simulink model "kde"  (R2022b)
settings: Solver=VariableStepAuto  StartTime=0.0  StopTime=orbit_E.T  RelTol=1e-9
values from neighbouring files (symbols this model uses):
  A0 = [1 0 0; 0 1 0; 0 0 1]    [test_script.m]
  earth_horizon = struct('dvst', 3*0.2 ,'accuracy', deg2rad(0.2))    [test_script.m]
  gyro = struct('c', 15e-3, 'ARW', 0.15, 'sigma_b', deg2rad(0.3) / 3600,                'freq', 262, 'accuracy', 2.4e-9)    [test_script.m]
  H0 = sqrt((-29615e-9)^2+(-1728e-9)^2+(5186e-9)^2)    [test_script.m]
  I = [Ix; Iy; Iz]    [test_script.m]
  Ir = 0.005    [test_script.m]
  K_d = 40 * Iz * 0.3 * orbit_E.n    [test_script.m]
  K_p = Iz * (20 * orbit_E.n)^2    [test_script.m]
  m_t = 5.9722e24    (= 5.9722e+24)    [test_script.m]
  Mr = 0    [test_script.m]
  orbit_E = struct('mu', astroConstants(13), 'a', astroConstants(23) + 2000,                    'e', 0.1, 'inc', deg2rad(10), 'G', astroConstants(1),                    'theta0', 0, 'R', astroConstants(23))    [test_script.m]
  orbit_S = struct('mu', astroConstants(4), 'a', astroConstants(2), 'e', 0.0167,                    'epsilon', deg2rad(23.45), 'G', astroConstants(1),                    'theta0', 0  )    [test_script.m]
  r = pos-pos_CG    [test_script.m]
  solarPanel = struct( 'r', r, 'P', radiation/(3e8),                      'rho_d', .1, 'rho_s', [.5, .5, .5, .5, .5 .5, .1, .1, .1, .1],                      'area', [.06 .06 .04 .06 .06 .04 .12 .12 .12 .12])    [test_script.m]
  sun_sensor = struct('dvst', 3*0.2 ,'accuracy', deg2rad(0.2))    [test_script.m]
  w0 = [0; 0; orbit_E.n]    [test_script.m]
  wr0 = 0    [test_script.m]
undefined symbols (not defined in the file or in its folder): a_e, e, e_e, inc, T_e, theta0, w_e
libraries: matrix_library x5, vrlib x3, simulink_extras x1, dspinverses x1
(part 1 of 2)
settings Model: Creator=stefa  LastModifiedBy=stefa
settings SolverCC: ZeroCrossAlgorithm=Adaptive

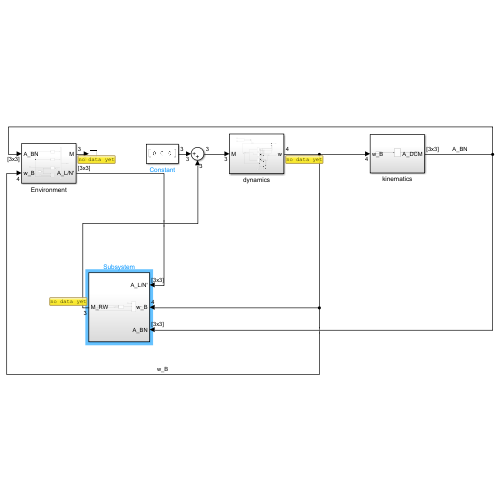
[thumbnail: Simulink's stored preview of the top-level diagram]
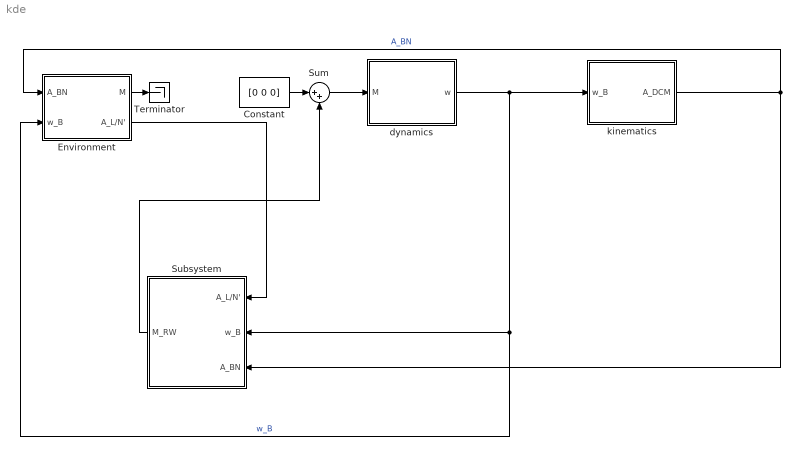
== system kde ==
  Constant : Constant  Value=[0 0 0]
  Environment : Subsystem
  Subsystem : Subsystem
  Sum : Sum  Inputs=|++
  Terminator : Terminator
  dynamics : Subsystem
  kinematics : Subsystem
  wires:
  dynamics/1(w) -> kinematics/1(w_B), Environment/2(w_B), Subsystem/2(w_B)  "w_B"
  kinematics/1(A_DCM) -> Environment/1(A_BN), Subsystem/3(A_BN)  "A_BN"
  Sum/1 -> dynamics/1(M)
  Environment/2(A_L/N') -> Subsystem/1(A_L/N')
  Subsystem/1(M_RW) -> Sum/2
  Constant/1 -> Sum/1
  Environment/1(M) -> Terminator/1

== system kde/Environment ==
  A_BN : Inport
  w_B : Inport  Port=2  PortDimensions=4
  Constant1 : Constant  Value=I
  Magnetic field : Subsystem
  Sum : Sum  Inputs=++++
  air drag : Subsystem  Commented=on
  gravity gradient : Subsystem
  inclination : Constant  Value=orbit_E.inc
  srp disturbance : Subsystem
  M : Outport
  A_L/N' : Outport  Port=2
  wires:
  A_BN/1 -> Magnetic field/1(A_BN), air drag/3(A_BN), gravity gradient/3(AB/N), srp disturbance/1(A_BN)
  Sum/1 -> M/1
  inclination/1 -> air drag/1(Inc), gravity gradient/2(inc)
  Constant1/1 -> gravity gradient/1(I)
  Magnetic field/1(M_B) -> Sum/1
  air drag/1(M_a) -> Sum/4
  w_B/1 -> air drag/2(w_B)
  srp disturbance/1(M_srp) -> Sum/2
  gravity gradient/1(M_g) -> Sum/3
  gravity gradient/2(A_L/N') -> A_L/N'/1

== system kde/Subsystem ==
  A_L/N' : Inport
  w_B : Inport  Port=2
  A_BN : Inport  Port=3
  Actuator : Subsystem
  Attitude Determination : Subsystem
  Sensors : Subsystem
  M_RW : Outport
  wires:
  w_B/1 -> Actuator/3(w_B), Sensors/1(w_B), Attitude Determination/3(v_B3)
  A_BN/1 -> Attitude Determination/2(A_mod)
  A_L/N'/1 -> Actuator/1(A_L/N')
  Attitude Determination/1(A_att) -> Actuator/2(A_B/N)
  Actuator/1(M_RW) -> M_RW/1
  Sensors/1(w_MB) -> Attitude Determination/1(s_Bgyro)

== system kde/dynamics ==
  M : Inport
  Constant1 : Constant  Value=I
  Constant3 : Constant  Value=Ir
  Constant4 : Constant  Value=Mr
  Constant5 : Constant  Value=w0
  Constant6 : Constant  Value=wr0
  Demux : Demux
  Demux1 : Demux  Outputs=3
  Demux2 : Demux  Outputs=3
  Integrator : Integrator  InitialConditionSource=external
  Mux : Mux  Inputs=3
  Mux1 : Mux  Inputs=2
  Mux2 : Mux  Inputs=2
  Product : Product  Inputs=*/
  Subsystem : Subsystem
  Subsystem1 : Subsystem
  Subsystem2 : Subsystem
  w : Outport
  wires:
  Constant1/1 -> Demux1/1
  Demux1/2 -> Subsystem/4(Iy), Subsystem1/4(Iy), Subsystem2/4(Iy)  "Iy"
  Integrator/1 -> w/1, Demux/1  "w"
  Demux1/1 -> Subsystem/3(Ix), Subsystem1/3(Ix), Subsystem2/3(Ix)  "Ix"
  Demux2/2 -> Subsystem1/6(My)  "My"
  Demux1/3 -> Subsystem/5(Iz), Subsystem1/5(Iz), Subsystem2/5(Iz)  "Iz"
  Subsystem1/1(wy_dot) -> Mux/2
  Demux/1 -> Subsystem1/1(wx), Subsystem2/1(wx)  "wx"
  Demux/4 -> Subsystem/8(wr), Subsystem1/8(wr)  "wr"
  Subsystem2/1(wz_dot) -> Mux/3
  Mux2/1 -> Integrator/2
  Demux2/3 -> Subsystem2/6(Mz)  "Mz"
  Constant6/1 -> Mux2/2
  M/1 -> Demux2/1
  Demux/3 -> Subsystem1/2(wz), Subsystem/2(wz)  "wz"
  Demux/2 -> Subsystem2/2(wy), Subsystem/1(wy)  "wy"
  Constant3/1 -> Product/2, Subsystem1/7(Ir), Subsystem/7(Ir), Subsystem2/7(Ir)
  Demux2/1 -> Subsystem/6(Mx)  "Mx"
  Mux1/1 -> Integrator/1  "w_dot, wr_dot"
  Product/1 -> Mux1/2, Subsystem2/8(wr_dot)  "wr_dot"
  Subsystem/1(wx_dot) -> Mux/1
  Constant5/1 -> Mux2/1
  Mux/1 -> Mux1/1  "w_dot"
  Constant4/1 -> Product/1

== system kde/kinematics ==
  w_B : Inport
  DCM : Subsystem
  A_DCM : Outport
  wires:
  w_B/1 -> DCM/1(w)
  DCM/1(A) -> A_DCM/1

== system kde/Environment/Magnetic field ==
  A_BN : Inport
  Cross Product : matrix_library/Cross Product
  Magnetic field : Subsystem
  m : Constant  Value=[0.01; 0.05; 0.01]
  M_B : Outport
  wires:
  A_BN/1 -> Magnetic field/1(A_BN)
  Magnetic field/1(b_B) -> Cross Product/2
  m/1 -> Cross Product/1
  Cross Product/1 -> M_B/1  "M_B"

== system kde/Environment/air drag ==
  Inc : Inport
  w_B : Inport  Port=2
  A_BN : Inport  Port=3
  Gain : Gain  Gain=-1
  MatrixMultiply : Product  Multiplication=Matrix(*)
  Selector : Selector  InputPortWidth=4  IndexOptions=Index vector (dialog)  Indices=[1 2 3]  OutputSizes=1
  Sum of Elements : Sum  Inputs=+
  air drag : Subsystem
  distance from the center of mass : Constant  Value=r
  M_a : Outport
  wires:
  MatrixMultiply/1 -> Sum of Elements/1
  Inc/1 -> air drag/1(Inc)
  air drag/1(F) -> MatrixMultiply/2
  Sum of Elements/1 -> Gain/1
  A_BN/1 -> air drag/2(A_BN)
  w_B/1 -> Selector/1
  Gain/1 -> M_a/1  "M_a"
  Selector/1 -> air drag/3(w_B)
  distance from the center of mass/1 -> MatrixMultiply/1, air drag/4(r)

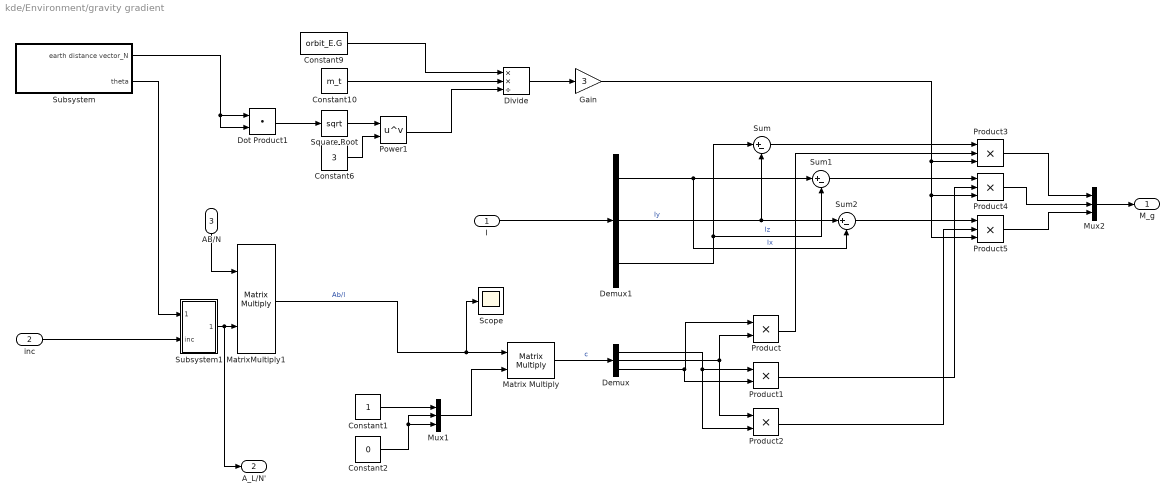
== system kde/Environment/gravity gradient ==
  I : Inport
  inc : Inport  Port=2
  AB/N : Inport  Port=3
  Constant1 : Constant
  Constant10 : Constant  Value=m_t
  Constant2 : Constant  Value=0
  Constant6 : Constant  Value=3
  Constant9 : Constant  Value=orbit_E.G
  Demux : Demux  Outputs=3
  Demux1 : Demux  Outputs=3
  Divide : Product  Inputs=**/
  Dot Product1 : DotProduct  OutDataTypeStr=Inherit: Inherit via internal rule
  Gain : Gain  Gain=3
  Matrix Multiply : Product  Multiplication=Matrix(*)
  MatrixMultiply1 : Product  Multiplication=Matrix(*)
  Mux1 : Mux  Inputs=3
  Mux2 : Mux  Inputs=3
  Power1 : Math  Operator=pow
  Product : Product
  Product1 : Product
  Product2 : Product
  Product3 : Product  Inputs=3
  Product4 : Product  Inputs=3
  Product5 : Product  Inputs=3
  Scope : Scope
  Square Root : Sqrt
  Subsystem : Subsystem
  Subsystem1 : Subsystem
  Sum : Sum  Inputs=|+-
  Sum1 : Sum  Inputs=|+-
  Sum2 : Sum  Inputs=|+-
  M_g : Outport
  A_L/N' : Outport  Port=2
  wires:
  AB/N/1 -> MatrixMultiply1/1
  MatrixMultiply1/1 -> Scope/1, Matrix Multiply/1  "Ab/l"
  Subsystem1/1(Al/n ') -> A_L/N'/1, MatrixMultiply1/2
  inc/1 -> Subsystem1/2(inc)
  Subsystem/2(theta) -> Subsystem1/1(theta)
  Product4/1 -> Mux2/2
  Gain/1 -> Product5/3, Product4/3, Product3/3
  Demux1/2 -> Sum/2, Sum2/1  "Iy"
  Demux/3 -> Product1/2, Product/1
  I/1 -> Demux1/1
  Divide/1 -> Gain/1
  Demux1/3 -> Sum/1, Sum1/2  "Iz"
  Product1/1 -> Product4/2
  Constant1/1 -> Mux1/1
  Sum2/1 -> Product5/1
  Square Root/1 -> Power1/1
  Matrix Multiply/1 -> Demux/1  "c"
  Constant9/1 -> Divide/1
  Sum/1 -> Product3/1
  Demux/2 -> Product/2, Product2/1
  Constant6/1 -> Power1/2
  Product3/1 -> Mux2/1
  Mux1/1 -> Matrix Multiply/2
  Product/1 -> Product3/2
  Constant10/1 -> Divide/2
  Demux1/1 -> Sum2/2, Sum1/1  "Ix"
  Product2/1 -> Product5/2
  Constant2/1 -> Mux1/3, Mux1/2
  Product5/1 -> Mux2/3
  Demux/1 -> Product2/2, Product1/1
  Sum1/1 -> Product4/1
  Power1/1 -> Divide/3
  Dot Product1/1 -> Square Root/1
  Mux2/1 -> M_g/1
  Subsystem/1(earth distance vector_N) -> Dot Product1/2, Dot Product1/1

== system kde/Environment/srp disturbance ==
  A_BN : Inport
  MatrixMultiply : Product  Multiplication=Matrix(*)
  Normalize Vector : vrlib/Utilities/Normalize Vector  maxzero=0
  Subsystem : Subsystem
  orientation s/c and solar panels : Subsystem
  sun distance magnitude : Subsystem
  M_srp : Outport
  wires:
  sun distance magnitude/1(S_N) -> Normalize Vector/1
  A_BN/1 -> MatrixMultiply/1
  Normalize Vector/1 -> MatrixMultiply/2
  Subsystem/1(M_SRP) -> M_srp/1
  orientation s/c and solar panels/1(N_B) -> Subsystem/2(N_B)
  MatrixMultiply/1 -> Subsystem/1(S_B)  "S_B"

== system kde/Subsystem/Actuator ==
  A_L/N' : Inport
  A_B/N : Inport  Port=2
  w_B : Inport  Port=3
  Constant : Constant  Value=I
  Display1 : Display
  IdentityMatrix : IdentityMatrix  OutputDimensions=3
  MatrixMultiply : Product  Multiplication=Matrix(*)
  Reaction wheels : Subsystem
  Subsystem : Subsystem
  state observer : Subsystem
  M_RW : Outport
  wires:
  IdentityMatrix/1 -> Reaction wheels/3(A)
  A_L/N'/1 -> MatrixMultiply/2
  w_B/1 -> state observer/1(y)
  Constant/1 -> state observer/2(I)
  MatrixMultiply/1 -> Display1/1, Subsystem/1(A_e)  "A_e"
  state observer/1(om) -> Reaction wheels/2(om), Subsystem/2(om)
  A_B/N/1 -> MatrixMultiply/1
  Subsystem/1(M_PD) -> state observer/3(Mc), Reaction wheels/1(M_PD)
  Reaction wheels/1(M_RW) -> M_RW/1

== system kde/Subsystem/Attitude Determination ==
  s_Bgyro : Inport
  A_mod : Inport  Port=2
  v_B3 : Inport  Port=3
  Constant : Constant  Value=sun_sensor.accuracy/(sun_sensor.accuracy + earth_horizon.accuracy + gyro.accuracy)
  Constant1 : Constant  Value=earth_horizon.accuracy/(sun_sensor.accuracy + earth_horizon.accuracy + gyro.accuracy)
  Constant2 : Constant  Value=gyro.accuracy/(sun_sensor.accuracy + earth_horizon.accuracy + gyro.accuracy)
  MATLAB Function : MATLAB Function  TreatAsAtomicUnit=on
  MatrixMultiply{,1..4} (5 alike) : Product  Multiplication=Matrix(*)
  Product1 : Product
  Product2 : Product
  Product3 : Product
  Selector : Selector  InputPortWidth=4  IndexOptions=Index vector (dialog)  Indices=[1 2 3]  OutputSizes=1
  Subsystem2 : Subsystem
  Sum : Sum  Inputs=+|+|+
  Transpose : Math  Operator=transpose
  A_att : Outport
  wires:
  MatrixMultiply/1 -> MatrixMultiply1/1
  MATLAB Function/1(U) -> MatrixMultiply/1
  MATLAB Function/2(M) -> MatrixMultiply/2
  MATLAB Function/3(V) -> Transpose/1
  Transpose/1 -> MatrixMultiply1/2
  MatrixMultiply1/1 -> A_att/1
  A_mod/1 -> Subsystem2/1(A_mod)
  Subsystem2/2(v_N1) -> MatrixMultiply3/2
  Subsystem2/1(s_B1) -> MatrixMultiply3/1
  Subsystem2/3(s_B2) -> MatrixMultiply4/1
  Subsystem2/4(v_N2) -> MatrixMultiply4/2
  MatrixMultiply4/1 -> Product1/1
  Constant1/1 -> Product1/2
  s_Bgyro/1 -> Subsystem2/2(s_Bgyro)
  v_B3/1 -> Selector/1
  Subsystem2/5(s_B3) -> MatrixMultiply2/1
  Subsystem2/6(v_N3) -> MatrixMultiply2/2
  MatrixMultiply2/1 -> Product2/1
  Constant2/1 -> Product2/2
  MatrixMultiply3/1 -> Product3/1
  Constant/1 -> Product3/2
  Product1/1 -> Sum/2
  Product2/1 -> Sum/3
  Product3/1 -> Sum/1
  Sum/1 -> MATLAB Function/1(B)
  Selector/1 -> Subsystem2/3(v_B3)

== system kde/Subsystem/Sensors ==
  w_B : Inport
  Constant : Constant  Value=gyro.c
  Constant1 : Constant  Value=gyro.A_eps
  MatrixMultiply1 : Product  Multiplication=Matrix(*)
  Product : Product
  Selector : Selector  InputPortWidth=4  IndexOptions=Index vector (dialog)  Indices=[1 2 3]  OutputSizes=1
  noise : Subsystem
  w_MB : Outport
  wires:
  MatrixMultiply1/1 -> noise/1(C*A*w_B)
  w_B/1 -> Selector/1
  Product/1 -> MatrixMultiply1/1
  Constant1/1 -> Product/2
  Constant/1 -> Product/1
  noise/1(w_M) -> w_MB/1
  Selector/1 -> MatrixMultiply1/2

== system kde/dynamics/Subsystem ==
  wy : Inport
  wz : Inport  Port=2
  Ix : Inport  Port=3
  Iy : Inport  Port=4
  Iz : Inport  Port=5
  Mx : Inport  Port=6
  Ir : Inport  Port=7
  wr : Inport  Port=8
  Product : Product
  Product1 : Product
  Product2 : Product  Inputs=3
  Product3 : Product  Inputs=*/
  Sum : Sum  Inputs=|+-
  Sum1 : Sum  Inputs=|+-+
  wx_dot : Outport
  wires:
  Product1/1 -> Sum1/1
  Product/1 -> Product1/1
  Product2/1 -> Sum1/2
  Ir/1 -> Product2/2
  Sum/1 -> Product1/2
  Product3/1 -> wx_dot/1  "wx_dot"
  Iy/1 -> Sum/1
  Iz/1 -> Sum/2
  wz/1 -> Product/1
  Mx/1 -> Sum1/3
  wy/1 -> Product2/1, Product/2
  Sum1/1 -> Product3/1
  Ix/1 -> Product3/2
  wr/1 -> Product2/3

== system kde/dynamics/Subsystem1 ==
  wx : Inport
  wz : Inport  Port=2
  Ix : Inport  Port=3
  Iy : Inport  Port=4
  Iz : Inport  Port=5
  My : Inport  Port=6
  Ir : Inport  Port=7
  wr : Inport  Port=8
  Product : Product
  Product1 : Product
  Product2 : Product  Inputs=3
  Product3 : Product  Inputs=*/
  Sum : Sum  Inputs=|+-
  Sum1 : Sum  Inputs=|++
  Sum2 : Sum  Inputs=|++
  wy_dot : Outport
  wires:
  Product1/1 -> Sum1/1
  Product2/1 -> Sum1/2
  Sum2/1 -> Product3/1
  Sum1/1 -> Sum2/1
  Iy/1 -> Product3/2
  Sum/1 -> Product1/2
  Iz/1 -> Sum/1
  Product/1 -> Product1/1
  Product3/1 -> wy_dot/1
  Ix/1 -> Sum/2
  My/1 -> Sum2/2
  wz/1 -> Product/1
  wx/1 -> Product2/1, Product/2
  wr/1 -> Product2/2
  Ir/1 -> Product2/3

== system kde/dynamics/Subsystem2 ==
  wx : Inport
  wy : Inport  Port=2
  Ix : Inport  Port=3
  Iy : Inport  Port=4
  Iz : Inport  Port=5
  Mz : Inport  Port=6
  Ir : Inport  Port=7
  wr_dot : Inport  Port=8
  Product : Product
  Product1 : Product
  Product2 : Product
  Product3 : Product  Inputs=*/
  Sum : Sum  Inputs=|+-
  Sum1 : Sum  Inputs=|+-+
  wz_dot : Outport
  wires:
  Sum/1 -> Product1/2
  Product/1 -> Product1/1
  Iz/1 -> Product3/2
  Product3/1 -> wz_dot/1  "wz_dot"
  Sum1/1 -> Product3/1
  Product2/1 -> Sum1/2
  Product1/1 -> Sum1/1
  Ix/1 -> Sum/1
  wy/1 -> Product/1
  Iy/1 -> Sum/2
  Mz/1 -> Sum1/3
  Ir/1 -> Product2/1
  wx/1 -> Product/2
  wr_dot/1 -> Product2/2

== system kde/kinematics/DCM ==
  w : Inport
  Constant : Constant  Value=0
  Constant1 : Constant  Value=A0
  Gain : Gain  Gain=3/2
  Gain1 : Gain  Gain=1/2
  Integrator : Integrator  InitialConditionSource=external
  MatrixMultiply : Product  Multiplication=Matrix(*)
  MatrixMultiply1 : Product  Inputs=3  Multiplication=Matrix(*)
  Selector : Selector  InputPortWidth=4  IndexOptions=Index vector (dialog)  Indices=[1 2 3]  OutputSizes=1
  Subsystem : Subsystem
  Sum : Sum  Inputs=|-+
  Transpose : Math  Operator=transpose
  A : Outport
  wires:
  Sum/1 -> A/1, MatrixMultiply/2
  Transpose/1 -> MatrixMultiply1/2
  MatrixMultiply/1 -> Integrator/1  "A_dot"
  Integrator/1 -> MatrixMultiply1/3, Gain/1, Transpose/1, MatrixMultiply1/1  "A"
  Subsystem/1(-[om^]) -> MatrixMultiply/1
  MatrixMultiply1/1 -> Gain1/1
  Constant/1 -> Subsystem/2(0)
  w/1 -> Selector/1
  Selector/1 -> Subsystem/1(w)
  Constant1/1 -> Integrator/2
  Gain1/1 -> Sum/1
  Gain/1 -> Sum/2

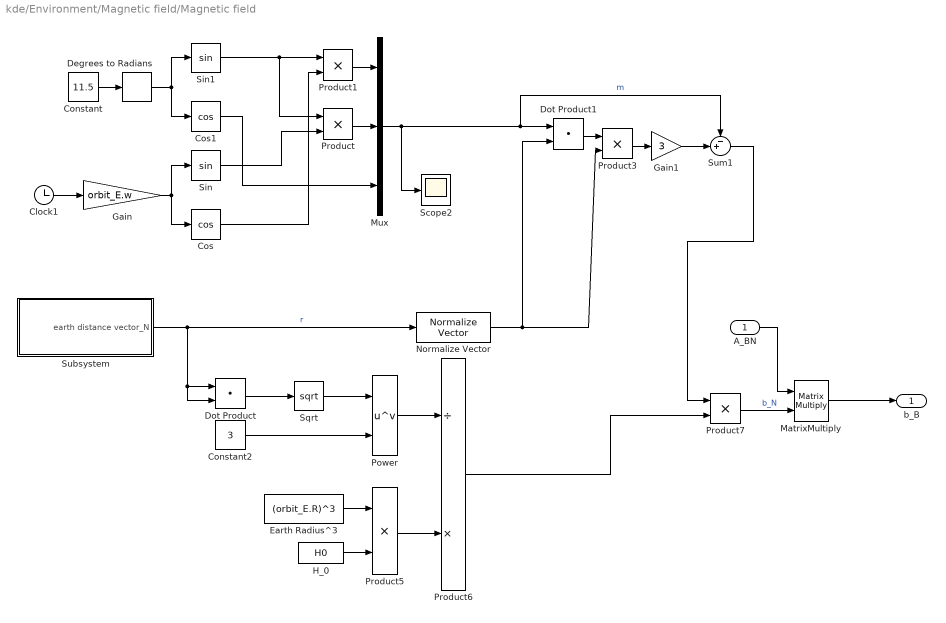
== system kde/Environment/Magnetic field/Magnetic field ==
  A_BN : Inport
  Clock1 : Clock
  Constant : Constant  Value=11.5
  Constant2 : Constant  Value=3
  Cos : Trigonometry  Operator=cos
  Cos1 : Trigonometry  Operator=cos
  Degrees to Radians : simulink_extras/Transformations/Degrees to Radians
  Dot Product : DotProduct  OutDataTypeStr=Inherit: Inherit via internal rule
  Dot Product1 : DotProduct  OutDataTypeStr=Inherit: Inherit via internal rule
  Earth Radius^3 : Constant  Value=(orbit_E.R)^3
  Gain : Gain  Gain=orbit_E.w
  Gain1 : Gain  Gain=3
  H_0 : Constant  Value=H0
  MatrixMultiply : Product  Multiplication=Matrix(*)
  Mux : Mux  Inputs=3
  Normalize Vector : vrlib/Utilities/Normalize Vector  maxzero=0
  Power : Math  Operator=pow
  Product{,1,3,5,7} (5 alike) : Product
  Product6 : Product  Inputs=/*
  Scope2 : Scope
  Sin : Trigonometry
  Sin1 : Trigonometry
  Sqrt : Sqrt
  Subsystem : Subsystem
  Sum1 : Sum  Inputs=-+|
  b_B : Outport
  wires:
  Constant2/1 -> Power/2
  Clock1/1 -> Gain/1
  Product1/1 -> Mux/1
  H_0/1 -> Product5/2
  Gain/1 -> Cos/1, Sin/1
  Subsystem/1(earth distance vector_N) -> Normalize Vector/1, Dot Product/1, Dot Product/2  "r"
  Mux/1 -> Dot Product1/1, Sum1/1, Scope2/1  "m"
  Dot Product/1 -> Sqrt/1
  Power/1 -> Product6/1
  Normalize Vector/1 -> Dot Product1/2, Product3/2
  Product6/1 -> Product7/2
  Dot Product1/1 -> Product3/1
  Product3/1 -> Gain1/1
  Degrees to Radians/1 -> Cos1/1, Sin1/1
  Cos1/1 -> Mux/3
  Product5/1 -> Product6/2
  Earth Radius^3/1 -> Product5/1
  Product/1 -> Mux/2
  Constant/1 -> Degrees to Radians/1
  Sin1/1 -> Product/1, Product1/1
  Sin/1 -> Product/2
  Product7/1 -> MatrixMultiply/2  "b_N"
  A_BN/1 -> MatrixMultiply/1
  MatrixMultiply/1 -> b_B/1
  Sqrt/1 -> Power/1
  Cos/1 -> Product1/2
  Sum1/1 -> Product7/1
  Gain1/1 -> Sum1/2

== system kde/Environment/air drag/air drag ==
  Inc : Inport
  A_BN : Inport  Port=2
  w_B : Inport  Port=3
  r : Inport  Port=4
  MATLAB Function : MATLAB Function  TreatAsAtomicUnit=on
  MatrixMultiply : Product  Multiplication=Matrix(*)
  Normalize Vector : vrlib/Utilities/Normalize Vector  maxzero=0
  Subsystem1 : Subsystem
  Subsystem11 : Subsystem
  Sum1 : Sum  Inputs=++|
  position vector : Subsystem
  true anomaly : Subsystem
  F : Outport
  wires:
  true anomaly/1(theta) -> Subsystem1/2(theta), position vector/1(theta)
  Subsystem1/1(vrel_N) -> MatrixMultiply/2
  MATLAB Function/1(y) -> Sum1/1
  MatrixMultiply/1 -> Sum1/2
  A_BN/1 -> MatrixMultiply/1
  Inc/1 -> Subsystem1/1(Inc)
  Sum1/1 -> Subsystem11/2(v_rel), Normalize Vector/1  "v_rel"
  Normalize Vector/1 -> Subsystem11/1(v_rel_1)
  Subsystem11/1(F) -> F/1
  w_B/1 -> MATLAB Function/1(w)
  r/1 -> MATLAB Function/2(r)
  position vector/1(R) -> Subsystem1/3(R)

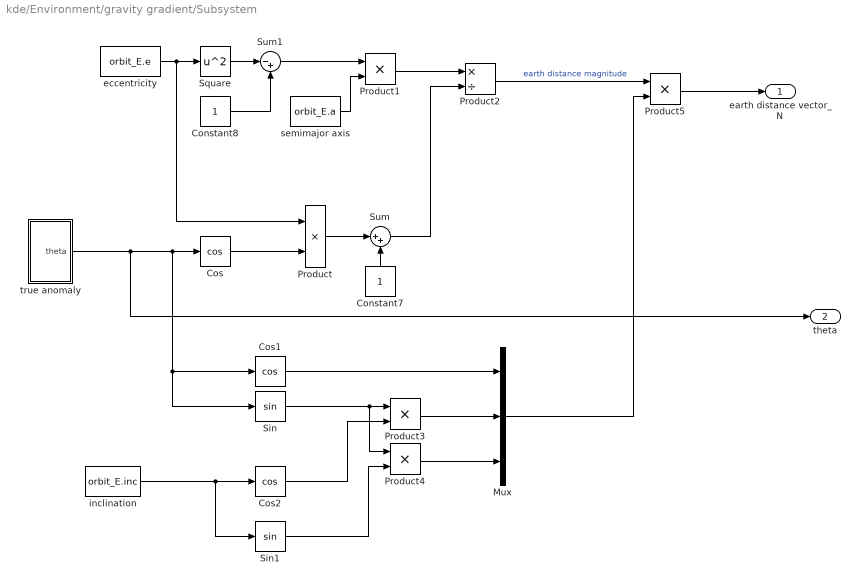
== system kde/Environment/gravity gradient/Subsystem ==
  Constant7 : Constant
  Constant8 : Constant
  Cos : Trigonometry  Operator=cos
  Cos1 : Trigonometry  Operator=cos
  Cos2 : Trigonometry  Operator=cos
  Mux : Mux  Inputs=3
  Product{,1,3..5} (5 alike) : Product
  Product2 : Product  Inputs=*/
  Sin : Trigonometry
  Sin1 : Trigonometry
  Square : Math  Operator=square
  Sum : Sum  Inputs=|++
  Sum1 : Sum  Inputs=|-+
  eccentricity : Constant  Value=orbit_E.e
  inclination : Constant  Value=orbit_E.inc
  semimajor axis : Constant  Value=orbit_E.a
  true anomaly : Subsystem
  earth distance vector_N : Outport
  theta : Outport  Port=2
  wires:
  Mux/1 -> Product5/2
  Product2/1 -> Product5/1  "earth distance magnitude"
  Product1/1 -> Product2/1
  Constant8/1 -> Sum1/2
  Sin/1 -> Product3/1, Product4/1
  true anomaly/1(theta) -> theta/1, Sin/1, Cos1/1, Cos/1
  Cos/1 -> Product/2
  eccentricity/1 -> Product/1, Square/1
  Sin1/1 -> Product4/2
  Sum1/1 -> Product1/1
  Sum/1 -> Product2/2
  Product3/1 -> Mux/2
  Cos1/1 -> Mux/1
  Square/1 -> Sum1/1
  semimajor axis/1 -> Product1/2
  inclination/1 -> Sin1/1, Cos2/1
  Product4/1 -> Mux/3
  Constant7/1 -> Sum/2
  Product/1 -> Sum/1
  Product5/1 -> earth distance vector_N/1
  Cos2/1 -> Product3/2

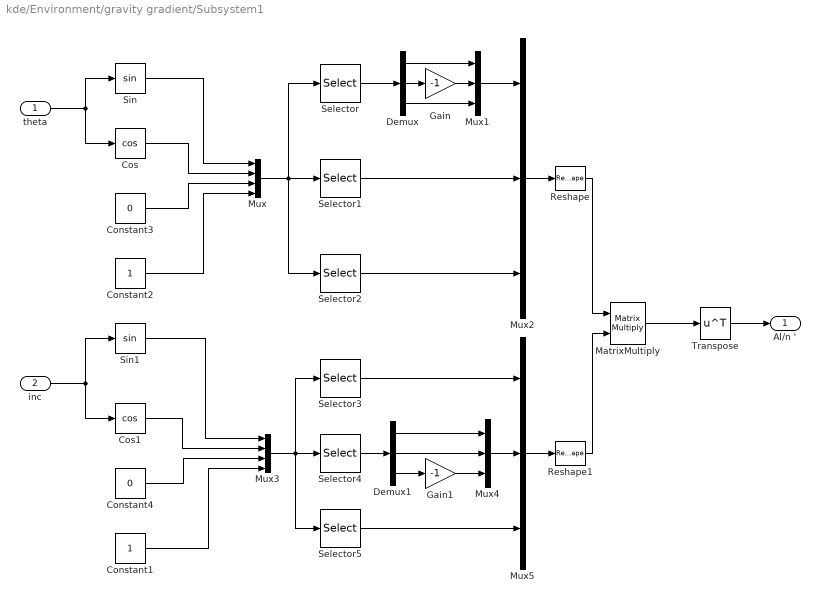
== system kde/Environment/gravity gradient/Subsystem1 ==
  theta : Inport
  inc : Inport  Port=2
  Constant1 : Constant
  Constant2 : Constant
  Constant3 : Constant  Value=0
  Constant4 : Constant  Value=0
  Cos : Trigonometry  Operator=cos
  Cos1 : Trigonometry  Operator=cos
  Demux : Demux  Outputs=3
  Demux1 : Demux  Outputs=3
  Gain : Gain  Gain=-1
  Gain1 : Gain  Gain=-1
  MatrixMultiply : Product  Multiplication=Matrix(*)
  Mux : Mux
  Mux{1..2,4..5} (4 alike) : Mux  Inputs=3
  Mux3 : Mux
  Reshape : Reshape  OutputDimensionality=Customize  OutputDimensions=[3,3]
  Reshape1 : Reshape  OutputDimensionality=Customize  OutputDimensions=[3,3]
  Selector : Selector  InputPortWidth=4  IndexOptions=Index vector (dialog)  Indices=[2 1 3]  OutputSizes=1
  Selector1 : Selector  InputPortWidth=4  IndexOptions=Index vector (dialog)  Indices=[1 2 3]  OutputSizes=1
  Selector2 : Selector  InputPortWidth=4  IndexOptions=Index vector (dialog)  Indices=[3 3 4]  OutputSizes=1
  Selector3 : Selector  InputPortWidth=4  IndexOptions=Index vector (dialog)  Indices=[4 3 3]  OutputSizes=1
  Selector4 : Selector  InputPortWidth=4  IndexOptions=Index vector (dialog)  Indices=[3 2 1]  OutputSizes=1
  Selector5 : Selector  InputPortWidth=4  IndexOptions=Index vector (dialog)  Indices=[3 1 2]  OutputSizes=1
  Sin : Trigonometry
  Sin1 : Trigonometry
  Transpose : Math  Operator=transpose
  Al/n ' : Outport
  wires:
  Constant2/1 -> Mux/4
  Constant3/1 -> Mux/3
  theta/1 -> Cos/1, Sin/1
  Cos/1 -> Mux/2
  Sin/1 -> Mux/1
  Mux/1 -> Selector2/1, Selector1/1, Selector/1
  Selector/1 -> Demux/1
  Demux/2 -> Gain/1
  Gain/1 -> Mux1/2
  Demux/3 -> Mux1/3
  Demux/1 -> Mux1/1
  Selector2/1 -> Mux2/3
  Mux1/1 -> Mux2/1
  Selector1/1 -> Mux2/2
  Mux2/1 -> Reshape/1
  Cos1/1 -> Mux3/2
  Sin1/1 -> Mux3/1
  Constant4/1 -> Mux3/3
  Constant1/1 -> Mux3/4
  inc/1 -> Cos1/1, Sin1/1
  Selector4/1 -> Demux1/1
  Demux1/3 -> Gain1/1
  Demux1/2 -> Mux4/2
  Demux1/1 -> Mux4/1
  Gain1/1 -> Mux4/3
  Mux3/1 -> Selector3/1, Selector4/1, Selector5/1
  Mux4/1 -> Mux5/2
  Selector3/1 -> Mux5/1
  Selector5/1 -> Mux5/3
  Mux5/1 -> Reshape1/1
  Reshape/1 -> MatrixMultiply/1
  Reshape1/1 -> MatrixMultiply/2
  MatrixMultiply/1 -> Transpose/1
  Transpose/1 -> Al/n '/1

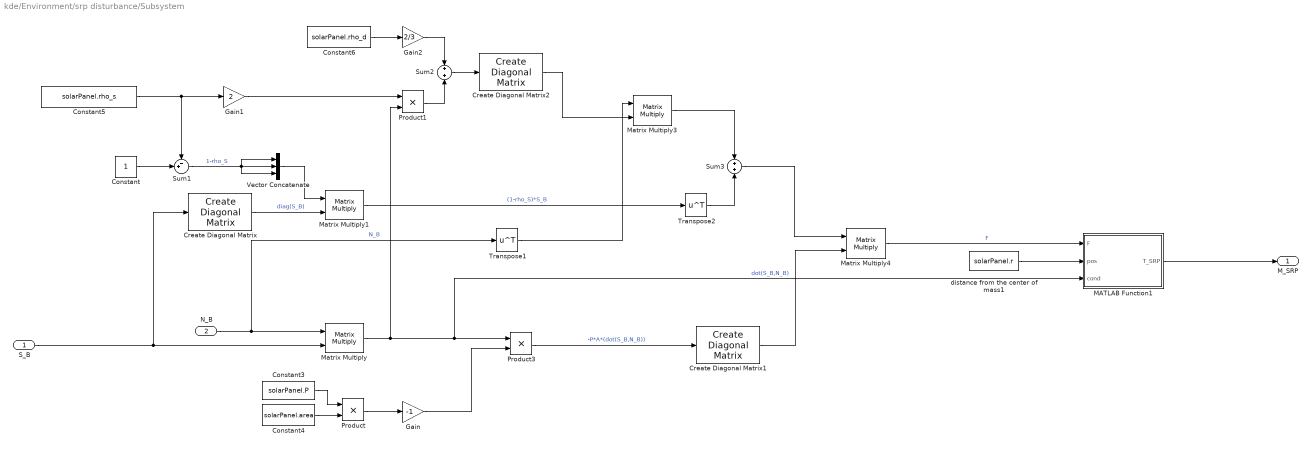
== system kde/Environment/srp disturbance/Subsystem ==
  S_B : Inport
  N_B : Inport  Port=2
  Constant : Constant
  Constant3 : Constant  Value=solarPanel.P
  Constant4 : Constant  Value=solarPanel.area
  Constant5 : Constant  Value=solarPanel.rho_s
  Constant6 : Constant  Value=solarPanel.rho_d
  Create Diagonal Matrix : matrix_library/Create Diagonal Matrix
      settings: LibrarySourceBlock=|
      | simulink/Matrix
      | Operations/Create Diagonal
      | Matrix
  Create Diagonal Matrix1 : matrix_library/Create Diagonal Matrix
      settings: LibrarySourceBlock=|
      | simulink/Matrix
      | Operations/Create Diagonal
      | Matrix
  Create Diagonal Matrix2 : matrix_library/Create Diagonal Matrix
      settings: LibrarySourceBlock=|
      | simulink/Matrix
      | Operations/Create Diagonal
      | Matrix
  Gain : Gain  Gain=-1
  Gain1 : Gain  Gain=2
  Gain2 : Gain  Gain=2/3
  MATLAB Function1 : MATLAB Function  TreatAsAtomicUnit=on
  Matrix Multiply{,1,3..4} (4 alike) : Product  Multiplication=Matrix(*)
  Product : Product
  Product1 : Product
  Product3 : Product
  Sum1 : Sum  Inputs=-+|
  Sum2 : Sum
  Sum3 : Sum
  Transpose1 : Math  Operator=transpose
  Transpose2 : Math  Operator=transpose
  Vector Concatenate : Concatenate  NumInputs=3  Mode=Multidimensional array  ConcatenateDimension=2
  distance from the center of mass1 : Constant  Value=solarPanel.r
  M_SRP : Outport
  wires:
  MATLAB Function1/1(T_SRP) -> M_SRP/1
  Create Diagonal Matrix1/1 -> Matrix Multiply4/2
  Product/1 -> Gain/1
  Matrix Multiply3/1 -> Sum3/1
  Product1/1 -> Sum2/2
  Transpose2/1 -> Sum3/2
  S_B/1 -> Create Diagonal Matrix/1, Matrix Multiply/2
  Constant4/1 -> Product/2
  Create Diagonal Matrix2/1 -> Matrix Multiply3/2
  Gain2/1 -> Sum2/1
  Constant/1 -> Sum1/2
  Matrix Multiply4/1 -> MATLAB Function1/1(F)  "F"
  Sum2/1 -> Create Diagonal Matrix2/1
  Product3/1 -> Create Diagonal Matrix1/1  "-P*A*(dot(S_B,N_B))"
  Create Diagonal Matrix/1 -> Matrix Multiply1/2  "diag(S_B)"
  N_B/1 -> Transpose1/1, Matrix Multiply/1  "N_B"
  Constant3/1 -> Product/1
  distance from the center of mass1/1 -> MATLAB Function1/2(pos)
  Matrix Multiply1/1 -> Transpose2/1  "(1-rho_S)*S_B"
  Constant5/1 -> Gain1/1, Sum1/1
  Gain/1 -> Product3/2
  Constant6/1 -> Gain2/1
  Sum1/1 -> Vector Concatenate/1, Vector Concatenate/3, Vector Concatenate/2  "1-rho_S"
  Gain1/1 -> Product1/1
  Sum3/1 -> Matrix Multiply4/1
  Matrix Multiply/1 -> Product1/2, MATLAB Function1/3(cond), Product3/1  "dot(S_B,N_B)"
  Vector Concatenate/1 -> Matrix Multiply1/1
  Transpose1/1 -> Matrix Multiply3/1

== system kde/Environment/srp disturbance/orientation s//c and solar panels ==
  Transpose : Math  Operator=transpose
  Vector Concatenate : Concatenate  NumInputs=10  Mode=Multidimensional array  ConcatenateDimension=2
  orientation s/c and solar panels in B : Subsystem
  N_B : Outport
  wires:
  orientation s/c and solar panels in B/6(n6) -> Vector Concatenate/6
  orientation s/c and solar panels in B/7(n7) -> Vector Concatenate/7
  orientation s/c and solar panels in B/3(n3) -> Vector Concatenate/3
  orientation s/c and solar panels in B/5(n5) -> Vector Concatenate/5
  orientation s/c and solar panels in B/10(n10) -> Vector Concatenate/10
  orientation s/c and solar panels in B/2(n2) -> Vector Concatenate/2
  orientation s/c and solar panels in B/8(n8) -> Vector Concatenate/8
  orientation s/c and solar panels in B/1(n1) -> Vector Concatenate/1
  orientation s/c and solar panels in B/4(n4) -> Vector Concatenate/4
  orientation s/c and solar panels in B/9(n9) -> Vector Concatenate/9
  Vector Concatenate/1 -> Transpose/1  "N_B"
  Transpose/1 -> N_B/1

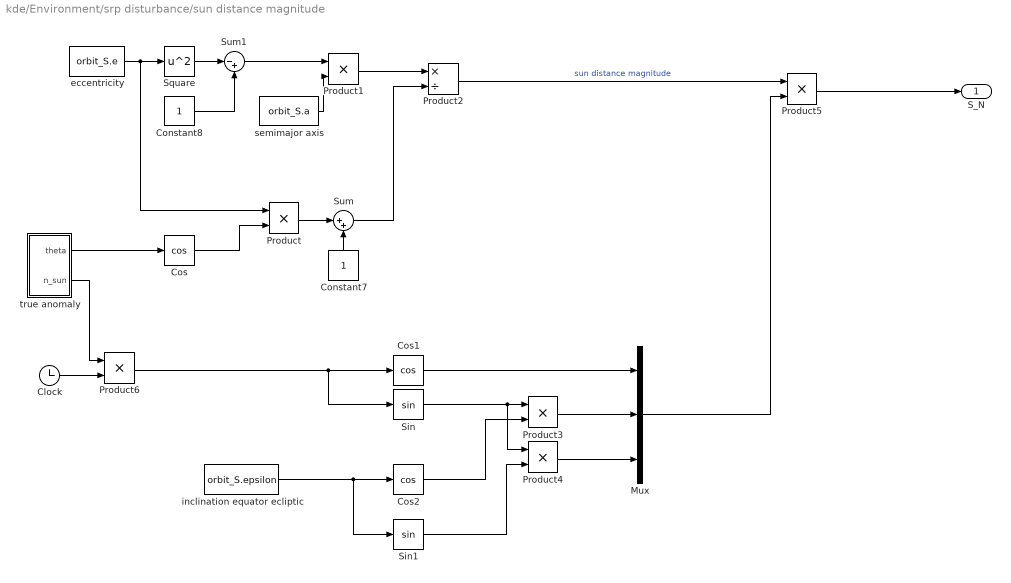
== system kde/Environment/srp disturbance/sun distance magnitude ==
  Clock : Clock
  Constant7 : Constant
  Constant8 : Constant
  Cos : Trigonometry  Operator=cos
  Cos1 : Trigonometry  Operator=cos
  Cos2 : Trigonometry  Operator=cos
  Mux : Mux  Inputs=3
  Product{,1,3..6} (6 alike) : Product
  Product2 : Product  Inputs=*/
  Sin : Trigonometry
  Sin1 : Trigonometry
  Square : Math  Operator=square
  Sum : Sum  Inputs=|++
  Sum1 : Sum  Inputs=|-+
  eccentricity : Constant  Value=orbit_S.e
  inclination equator ecliptic : Constant  Value=orbit_S.epsilon
  semimajor axis : Constant  Value=orbit_S.a
  true anomaly : Subsystem
  S_N : Outport
  wires:
  Mux/1 -> Product5/2
  Product2/1 -> Product5/1  "sun distance magnitude"
  Product1/1 -> Product2/1
  Constant8/1 -> Sum1/2
  Sin/1 -> Product4/1, Product3/1
  Cos/1 -> Product/2
  eccentricity/1 -> Product/1, Square/1
  Sin1/1 -> Product4/2
  Sum1/1 -> Product1/1
  Product3/1 -> Mux/2
  Cos1/1 -> Mux/1
  Square/1 -> Sum1/1
  semimajor axis/1 -> Product1/2
  inclination equator ecliptic/1 -> Sin1/1, Cos2/1
  Product4/1 -> Mux/3
  Constant7/1 -> Sum/2
  Product/1 -> Sum/1
  Cos2/1 -> Product3/2
  true anomaly/1(theta) -> Cos/1
  Clock/1 -> Product6/2
  true anomaly/2(n_sun) -> Product6/1
  Product6/1 -> Sin/1, Cos1/1
  Sum/1 -> Product2/2
  Product5/1 -> S_N/1

== system kde/Subsystem/Actuator/Reaction wheels ==
  M_PD : Inport
  om : Inport  Port=2
  A : Inport  Port=3
  RW dynamics : Subsystem
  M_RW : Outport
  wires:
  M_PD/1 -> RW dynamics/1(M_PD)
  om/1 -> RW dynamics/2(om)
  A/1 -> RW dynamics/3(A)
  RW dynamics/1(hr_dot) -> M_RW/1

== system kde/Subsystem/Actuator/Subsystem ==
  A_e : Inport
  om : Inport  Port=2
  Constant : Constant  Value=K_d
  Constant1 : Constant  Value=K_p
  Demux : Demux  Outputs=9
  Gain : Gain  Gain=1/2
  Mux : Mux  Inputs=3
  Product : Product
  Product1 : Product
  Reshape : Reshape  OutputDimensionality=Column vector (2-D)
  Sum : Sum  Inputs=-+|
  Sum1 : Sum  Inputs=|+-
  Sum2 : Sum  Inputs=|-+
  Sum3 : Sum  Inputs=+|+
  Terminator : Terminator
  Terminator1 : Terminator
  Terminator2 : Terminator
  M_PD : Outport
  wires:
  Constant/1 -> Product/1
  om/1 -> Product/2
  Constant1/1 -> Gain/1
  A_e/1 -> Reshape/1
  Reshape/1 -> Demux/1
  Demux/1 -> Terminator2/1  "a11"
  Demux/2 -> Sum/1  "a21"
  Demux/3 -> Sum1/1  "a31"
  Demux/4 -> Sum/2  "a12"
  Demux/5 -> Terminator1/1  "a22"
  Demux/6 -> Sum2/1  "a32"
  Demux/7 -> Sum1/2  "a13"
  Demux/8 -> Sum2/2  "a23"
  Demux/9 -> Terminator/1  "a33"
  Sum1/1 -> Mux/2
  Sum2/1 -> Mux/1
  Sum/1 -> Mux/3
  Mux/1 -> Product1/2
  Gain/1 -> Product1/1
  Product1/1 -> Sum3/1
  Product/1 -> Sum3/2
  Sum3/1 -> M_PD/1

== system kde/Subsystem/Actuator/state observer ==
  y : Inport
  I : Inport  Port=2
  Mc : Inport  Port=3
  Constant : Constant  Value=orbit_E.n
  Constant1 : Constant  Value=zeros(6, 1)
  Integrator : Integrator  InitialConditionSource=external
  MATLAB Function : MATLAB Function  TreatAsAtomicUnit=on
  MatrixMultiply1 : Product  Multiplication=Matrix(*)
  MatrixMultiply2 : Product  Multiplication=Matrix(*)
  Selector : Selector  InputPortWidth=4  IndexOptions=Index vector (dialog)  Indices=[1 2 3]  OutputSizes=1
  Subsystem : Subsystem
  Subsystem1 : Subsystem
  Sum : Sum  Inputs=+|+|+
  om : Outport
  wires:
  Sum/1 -> Integrator/1  "alha_dot"
  Integrator/1 -> Subsystem1/1(alpha), Subsystem/1(alpha)  "alpha"
  Mc/1 -> MatrixMultiply1/2
  Subsystem/1(om_B) -> om/1
  Subsystem1/1(L) -> MatrixMultiply2/1
  MatrixMultiply1/1 -> Sum/3
  MatrixMultiply2/1 -> Sum/1
  Subsystem1/2(A_hat*alpha) -> Sum/2
  Selector/1 -> MatrixMultiply2/2
  y/1 -> Selector/1
  Constant1/1 -> Integrator/2
  I/1 -> MATLAB Function/1(I)
  Constant/1 -> MATLAB Function/2(n)
  MATLAB Function/1(A) -> Subsystem1/2(A)
  MATLAB Function/2(C) -> Subsystem1/3(C)
  MATLAB Function/3(B) -> MatrixMultiply1/1, Subsystem1/4(B)  "B"

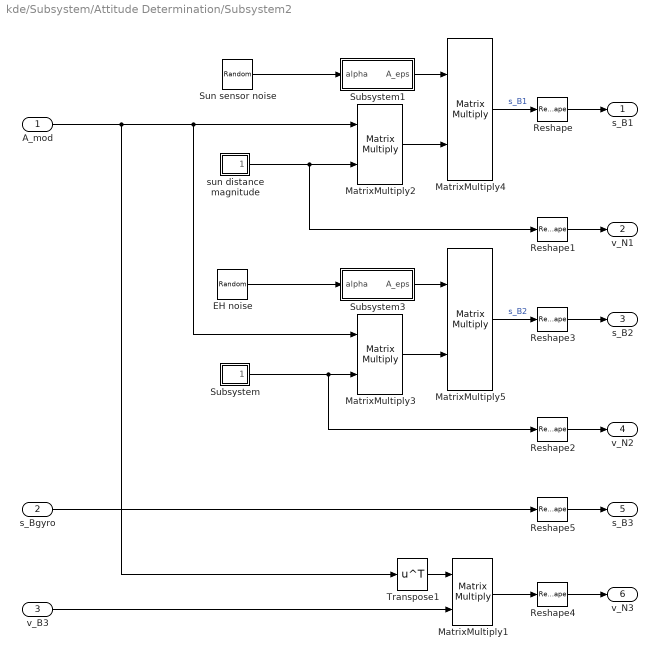
== system kde/Subsystem/Attitude Determination/Subsystem2 ==
  A_mod : Inport
  s_Bgyro : Inport  Port=2
  v_B3 : Inport  Port=3
  EH noise : RandomNumber  Variance=(deg2rad(earth_horizon.dvst))^2  SampleTime=0.1
  MatrixMultiply{1..5} (5 alike) : Product  Multiplication=Matrix(*)
  Reshape : Reshape  OutputDimensionality=Column vector (2-D)
  Reshape1 : Reshape  OutputDimensionality=Row vector (2-D)
  Reshape2 : Reshape  OutputDimensionality=Row vector (2-D)
  Reshape3 : Reshape  OutputDimensionality=Column vector (2-D)
  Reshape4 : Reshape  OutputDimensionality=Row vector (2-D)
  Reshape5 : Reshape  OutputDimensionality=Column vector (2-D)
  Subsystem : Subsystem
  Subsystem1 : Subsystem
  Subsystem3 : Subsystem
  Sun sensor noise : RandomNumber  Variance=(deg2rad(sun_sensor.dvst))^2  SampleTime=0.1
  Transpose1 : Math  Operator=transpose
  sun distance magnitude : Subsystem
  s_B1 : Outport
  v_N1 : Outport  Port=2
  s_B2 : Outport  Port=3
  v_N2 : Outport  Port=4
  s_B3 : Outport  Port=5
  v_N3 : Outport  Port=6
  wires:
  EH noise/1 -> Subsystem3/1(alpha)
  Subsystem/1(R_N) -> Reshape2/1, MatrixMultiply3/2
  Subsystem3/1(A_eps) -> MatrixMultiply5/1
  Subsystem1/1(A_eps) -> MatrixMultiply4/1
  MatrixMultiply3/1 -> MatrixMultiply5/2
  Sun sensor noise/1 -> Subsystem1/1(alpha)
  MatrixMultiply4/1 -> Reshape/1  "s_B1"
  MatrixMultiply2/1 -> MatrixMultiply4/2
  sun distance magnitude/1(S_N) -> Reshape1/1, MatrixMultiply2/2
  MatrixMultiply5/1 -> Reshape3/1  "s_B2"
  Reshape/1 -> s_B1/1
  Reshape1/1 -> v_N1/1
  Reshape2/1 -> v_N2/1
  Reshape3/1 -> s_B2/1
  MatrixMultiply1/1 -> Reshape4/1
  A_mod/1 -> Transpose1/1, MatrixMultiply2/1, MatrixMultiply3/1
  v_B3/1 -> MatrixMultiply1/2
  Transpose1/1 -> MatrixMultiply1/1
  Reshape4/1 -> v_N3/1
  s_Bgyro/1 -> Reshape5/1
  Reshape5/1 -> s_B3/1

== system kde/Subsystem/Sensors/noise ==
  C*A*w_B : Inport
  Integrator : Integrator
  Sum : Sum  Inputs=+++
  b_dot : RandomNumber  Variance=(gyro.sigma_b) ^2  SampleTime=1/gyro.freq
  n : RandomNumber  Variance=(deg2rad(gyro.ARW)/60 * sqrt(gyro.freq))^2  SampleTime=1/gyro.freq
  w_M : Outport
  wires:
  b_dot/1 -> Integrator/1
  Sum/1 -> w_M/1
  n/1 -> Sum/2
  Integrator/1 -> Sum/3  "b"
  C*A*w_B/1 -> Sum/1

== system kde/kinematics/DCM/Subsystem ==
  w : Inport
  0 : Inport  Port=2
  Demux : Demux  Outputs=3
  Demux1 : Demux  Outputs=3
  Demux2 : Demux  Outputs=3
  Gain : Gain  Gain=-1
  Gain1 : Gain  Gain=-1
  Gain2 : Gain  Gain=-1
  Matrix Concatenate : Concatenate  NumInputs=3  Mode=Multidimensional array  ConcatenateDimension=2
  Mux : Mux  Inputs=2
  Mux1 : Mux  Inputs=3
  Mux2 : Mux  Inputs=3
  Mux3 : Mux  Inputs=3
  Selector : Selector  InputPortWidth=4  IndexOptions=Index vector (dialog)  Indices=[4 3 2]  OutputSizes=1
  Selector1 : Selector  InputPortWidth=4  IndexOptions=Index vector (dialog)  Indices=[3 4 1]  OutputSizes=1
  Selector2 : Selector  InputPortWidth=4  IndexOptions=Index vector (dialog)  Indices=[2 1 4]  OutputSizes=1
  -[om^] : Outport
  wires:
  w/1 -> Mux/1
  Demux/3 -> Mux1/3
  Demux/1 -> Mux1/1
  Demux2/3 -> Mux3/3
  Selector2/1 -> Demux2/1
  Mux/1 -> Selector2/1, Selector1/1, Selector/1
  Selector/1 -> Demux/1
  Demux/2 -> Gain/1
  Mux3/1 -> Matrix Concatenate/3
  Mux1/1 -> Matrix Concatenate/1
  Demux2/2 -> Mux3/2
  Gain1/1 -> Mux2/3
  Selector1/1 -> Demux1/1
  Demux1/2 -> Mux2/2
  Demux1/3 -> Gain1/1
  Gain/1 -> Mux1/2
  Mux2/1 -> Matrix Concatenate/2
  Demux1/1 -> Mux2/1
  Demux2/1 -> Gain2/1
  Gain2/1 -> Mux3/1
  Matrix Concatenate/1 -> -[om^]/1
  0/1 -> Mux/2

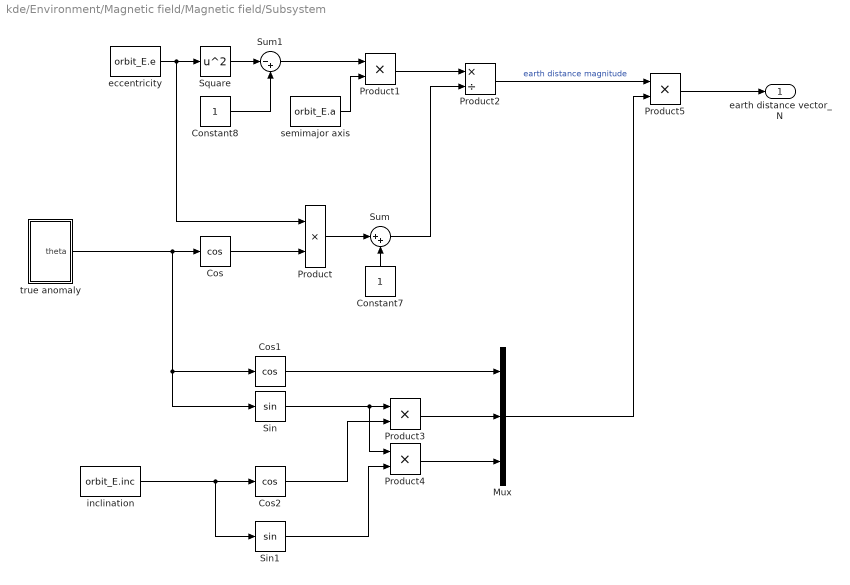
== system kde/Environment/Magnetic field/Magnetic field/Subsystem ==
  Constant7 : Constant
  Constant8 : Constant
  Cos : Trigonometry  Operator=cos
  Cos1 : Trigonometry  Operator=cos
  Cos2 : Trigonometry  Operator=cos
  Mux : Mux  Inputs=3
  Product{,1,3..5} (5 alike) : Product
  Product2 : Product  Inputs=*/
  Sin : Trigonometry
  Sin1 : Trigonometry
  Square : Math  Operator=square
  Sum : Sum  Inputs=|++
  Sum1 : Sum  Inputs=|-+
  eccentricity : Constant  Value=orbit_E.e
  inclination : Constant  Value=orbit_E.inc
  semimajor axis : Constant  Value=orbit_E.a
  true anomaly : Subsystem
  earth distance vector_N : Outport
  wires:
  Mux/1 -> Product5/2
  Product2/1 -> Product5/1  "earth distance magnitude"
  Product1/1 -> Product2/1
  Constant8/1 -> Sum1/2
  Sin/1 -> Product3/1, Product4/1
  true anomaly/1(theta) -> Sin/1, Cos1/1, Cos/1
  Cos/1 -> Product/2
  eccentricity/1 -> Product/1, Square/1
  Sin1/1 -> Product4/2
  Sum1/1 -> Product1/1
  Sum/1 -> Product2/2
  Product3/1 -> Mux/2
  Cos1/1 -> Mux/1
  Square/1 -> Sum1/1
  semimajor axis/1 -> Product1/2
  inclination/1 -> Sin1/1, Cos2/1
  Product4/1 -> Mux/3
  Constant7/1 -> Sum/2
  Product/1 -> Sum/1
  Product5/1 -> earth distance vector_N/1
  Cos2/1 -> Product3/2

== system kde/Environment/air drag/air drag/Subsystem1 ==
  Inc : Inport
  theta : Inport  Port=2
  R : Inport  Port=3
  Demux : Demux  Outputs=3
  Demux1 : Demux  Outputs=3
  Display : Display
  Display1 : Display
  Dot Product : DotProduct  OutDataTypeStr=Inherit: Inherit via internal rule
  Gain : Gain  Gain=w_e
  Mux : Mux  Inputs=3
  Product1 : Product
  Sqrt : Sqrt
  Subsystem : Subsystem
  Sum1 : Sum  Inputs=|++
  Sum2 : Sum  Inputs=|+-
  vrel_N : Outport
  wires:
  Gain/1 -> Demux1/1
  Product1/1 -> Gain/1, Display1/1, Demux/1, Display/1  "[x y z]"
  Demux/2 -> Sum2/1
  Mux/1 -> vrel_N/1  "vrel_b"
  Demux/1 -> Sum1/1
  R/1 -> Dot Product/2, Dot Product/1
  Sum1/1 -> Mux/1
  Demux1/1 -> Sum2/2
  Demux1/2 -> Sum1/2
  Subsystem/1(Out1) -> Product1/1
  Demux/3 -> Mux/3
  Sum2/1 -> Mux/2
  Inc/1 -> Subsystem/1(Inc)
  theta/1 -> Subsystem/2(theta)
  Dot Product/1 -> Sqrt/1
  Sqrt/1 -> Product1/2  "R_norm"

== system kde/Environment/air drag/air drag/Subsystem11 ==
  v_rel_1 : Inport
  v_rel : Inport  Port=2
  Display : Display
  Display1 : Display
  MATLAB Function : MATLAB Function  TreatAsAtomicUnit=on
  orientation s/c and solar panels : Subsystem
  F : Outport
  wires:
  MATLAB Function/1(y) -> F/1
  v_rel_1/1 -> Display1/1, MATLAB Function/1(v_rel_1)
  orientation s/c and solar panels/1(N_B) -> MATLAB Function/2(N), Display/1
  v_rel/1 -> MATLAB Function/3(v_rel)

== system kde/Environment/air drag/air drag/position vector ==
  theta : Inport
  Constant7 : Constant
  Constant8 : Constant
  Cos : Trigonometry  Operator=cos
  Cos1 : Trigonometry  Operator=cos
  Cos2 : Trigonometry  Operator=cos
  Mux : Mux  Inputs=3
  Product{,1,3..5} (5 alike) : Product
  Product2 : Product  Inputs=*/
  Sin : Trigonometry
  Sin1 : Trigonometry
  Square : Math  Operator=square
  Sum : Sum  Inputs=|++
  Sum1 : Sum  Inputs=|+-
  eccentricity : Constant  Value=e_e
  inclination : Constant  Value=inc
  semimajor axis : Constant  Value=a_e
  R : Outport
  wires:
  Product5/1 -> R/1
  Cos2/1 -> Product3/2
  Product3/1 -> Mux/2
  Sum1/1 -> Product1/1
  Product/1 -> Sum/1
  Square/1 -> Sum1/1
  theta/1 -> Sin/1, Cos1/1, Cos/1
  Cos1/1 -> Mux/1
  Sum/1 -> Product2/2
  Cos/1 -> Product/2
  Sin1/1 -> Product4/2
  Constant7/1 -> Sum/2
  Sin/1 -> Product4/1, Product3/1
  inclination/1 -> Sin1/1, Cos2/1
  Constant8/1 -> Sum1/2
  Product1/1 -> Product2/1
  Product2/1 -> Product5/1  "earth distance magnitude"
  eccentricity/1 -> Product/1, Square/1
  semimajor axis/1 -> Product1/2
  Mux/1 -> Product5/2
  Product4/1 -> Mux/3

== system kde/Environment/air drag/air drag/true anomaly ==
  Constant : Constant  Value=theta0
  Constant10 : Constant  Value=3/2
  Constant7 : Constant  Value=2*pi
  Constant8 : Constant
  Constant9 : Constant
  Cos : Trigonometry  Operator=cos
  Integrator : Integrator  InitialConditionSource=external
  Power : Math  Operator=pow
  Product : Product  Inputs=*/
  Product1 : Product
  Product2 : Product
  Product3 : Product  Inputs=/*
  Square : Math  Operator=square
  Square1 : Math  Operator=square
  Sum : Sum  Inputs=|++
  Sum1 : Sum  Inputs=|-+
  eccentricity : Constant  Value=e
  period around the earth : Constant  Value=T_e
  theta : Outport
  wires:
  Sum/1 -> Square/1
  Product1/1 -> Sum/1
  Constant7/1 -> Product/1
  Integrator/1 -> theta/1, Cos/1  "theta"
  Cos/1 -> Product1/1
  Square/1 -> Product2/1
  period around the earth/1 -> Product/2
  Constant8/1 -> Sum/2
  Square1/1 -> Sum1/1
  eccentricity/1 -> Square1/1, Product1/2
  Constant10/1 -> Power/2
  Product/1 -> Product2/2
  Sum1/1 -> Power/1
  Constant9/1 -> Sum1/2
  Power/1 -> Product3/2
  Product3/1 -> Integrator/1  "theta_dot"
  Product2/1 -> Product3/1
  Constant/1 -> Integrator/2

== system kde/Environment/gravity gradient/Subsystem/true anomaly ==
  Constant : Constant  Value=orbit_E.theta0
  Constant1 : Constant  Value=orbit_E.n
  Constant10 : Constant  Value=3/2
  Constant8 : Constant
  Constant9 : Constant
  Cos : Trigonometry  Operator=cos
  Integrator : Integrator  InitialConditionSource=external
  Power : Math  Operator=pow
  Product1 : Product
  Product2 : Product
  Product3 : Product  Inputs=*/
  Square : Math  Operator=square
  Square1 : Math  Operator=square
  Sum : Sum  Inputs=|++
  Sum1 : Sum  Inputs=|-+
  eccentricity : Constant  Value=orbit_E.e
  theta : Outport
  wires:
  eccentricity/1 -> Square1/1, Product1/2
  Sum1/1 -> Power/1
  Product3/1 -> Integrator/1  "theta_dot"
  Constant9/1 -> Sum1/2
  Constant8/1 -> Sum/2
  Square1/1 -> Sum1/1
  Square/1 -> Product2/1
  Sum/1 -> Square/1
  Product2/1 -> Product3/1
  Cos/1 -> Product1/1
  Power/1 -> Product3/2
  Constant10/1 -> Power/2
  Integrator/1 -> theta/1, Cos/1  "theta"
  Constant/1 -> Integrator/2
  Product1/1 -> Sum/1
  Constant1/1 -> Product2/2

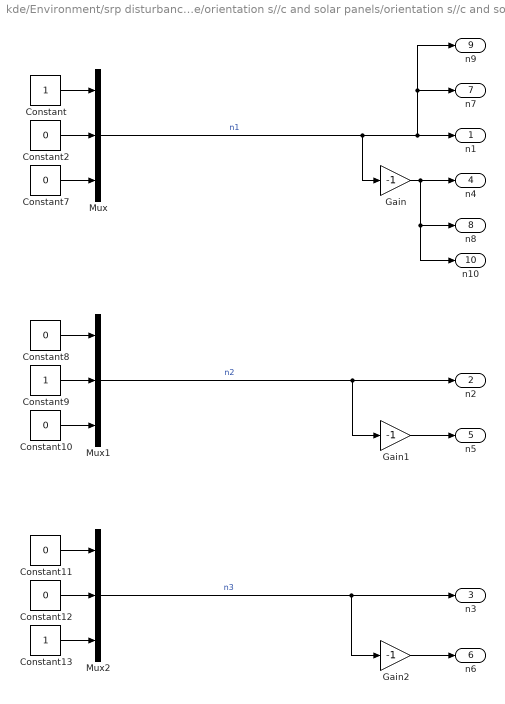
== system kde/Environment/srp disturbance/orientation s//c and solar panels/orientation s//c and solar panels in B ==
  Constant : Constant
  Constant{2,7..8,10..12} (6 alike) : Constant  Value=0
  Constant13 : Constant
  Constant9 : Constant
  Gain : Gain  Gain=-1
  Gain1 : Gain  Gain=-1
  Gain2 : Gain  Gain=-1
  Mux : Mux  Inputs=3
  Mux1 : Mux  Inputs=3
  Mux2 : Mux  Inputs=3
  n1 : Outport
  n2 : Outport  Port=2
  n3 : Outport  Port=3
  n4 : Outport  Port=4
  n5 : Outport  Port=5
  n6 : Outport  Port=6
  n7 : Outport  Port=7
  n8 : Outport  Port=8
  n9 : Outport  Port=9
  n10 : Outport  Port=10
  wires:
  Mux1/1 -> Gain1/1, n2/1  "n2"
  Mux2/1 -> n3/1, Gain2/1  "n3"
  Constant7/1 -> Mux/3
  Constant9/1 -> Mux1/2
  Gain1/1 -> n5/1
  Gain/1 -> n10/1, n8/1, n4/1
  Mux/1 -> Gain/1, n9/1, n7/1, n1/1  "n1"
  Constant11/1 -> Mux2/1
  Constant12/1 -> Mux2/2
  Gain2/1 -> n6/1
  Constant13/1 -> Mux2/3
  Constant10/1 -> Mux1/3
  Constant2/1 -> Mux/2
  Constant/1 -> Mux/1
  Constant8/1 -> Mux1/1

== system kde/Environment/srp disturbance/sun distance magnitude/true anomaly ==
  Constant : Constant  Value=orbit_S.theta0
  Constant1 : Constant  Value=orbit_S.n
  Constant10 : Constant  Value=3/2
  Constant8 : Constant
  Constant9 : Constant
  Cos : Trigonometry  Operator=cos
  Integrator : Integrator  InitialConditionSource=external
  Power : Math  Operator=pow
  Product1 : Product
  Product2 : Product
  Product3 : Product  Inputs=*/
  Square : Math  Operator=square
  Square1 : Math  Operator=square
  Sum : Sum  Inputs=|++
  Sum1 : Sum  Inputs=|-+
  eccentricity : Constant  Value=orbit_S.e
  theta : Outport
  n_sun : Outport  Port=2
  wires:
  Sum/1 -> Square/1
  Product1/1 -> Sum/1
  Integrator/1 -> theta/1, Cos/1  "theta"
  Cos/1 -> Product1/1
  Square/1 -> Product2/1
  Constant8/1 -> Sum/2
  Square1/1 -> Sum1/1
  eccentricity/1 -> Square1/1, Product1/2
  Constant10/1 -> Power/2
  Sum1/1 -> Power/1
  Constant9/1 -> Sum1/2
  Power/1 -> Product3/2
  Product3/1 -> Integrator/1  "theta_dot"
  Product2/1 -> Product3/1
  Constant/1 -> Integrator/2
  Constant1/1 -> n_sun/1, Product2/2

== system kde/Subsystem/Actuator/Reaction wheels/RW dynamics ==
  M_PD : Inport
  om : Inport  Port=2
  A : Inport  Port=3
  Cross Product : matrix_library/Cross Product
  Gain : Gain  Gain=-1
  Integrator : Integrator
  MatrixMultiply : Product  Multiplication=Matrix(*)
  MatrixMultiply1 : Product  Multiplication=Matrix(*)
  Pseudoinverse : dspinverses/Pseudoinverse  wanterr=off  SimulateUsing=Interpreted execution
  Sum : Sum  Inputs=|++
  hr_dot : Outport
  wires:
  A/1 -> MatrixMultiply/1, Pseudoinverse/1
  Integrator/1 -> MatrixMultiply/2  "hr"
  Gain/1 -> hr_dot/1, Integrator/1  "hr_dot"
  M_PD/1 -> Sum/2
  Pseudoinverse/1 -> MatrixMultiply1/1
  Sum/1 -> MatrixMultiply1/2
  MatrixMultiply1/1 -> Gain/1
  MatrixMultiply/1 -> Cross Product/2
  Cross Product/1 -> Sum/1
  om/1 -> Cross Product/1

== system kde/Subsystem/Actuator/state observer/Subsystem ==
  alpha : Inport
  Constant : Constant
  Constant1 : Constant
  Constant2 : Constant
  Constant3 : Constant  Value="[0  0 orbit_E.n]"
  Demux : Demux  Outputs=6
  Demux1 : Demux  Outputs=3
  Gain1 : Gain  Gain=-1
  Gain2 : Gain  Gain=-1
  Gain3 : Gain  Gain=-1
  MatrixMultiply3 : Product  Multiplication=Matrix(*)
  Mux{,1..5} (6 alike) : Mux  Inputs=3
  Reshape : Reshape  OutputDimensionality=Customize  OutputDimensions=[3,3]
  Sum1 : Sum  Inputs=++|
  om_B : Outport
  wires:
  Constant1/1 -> Mux2/1
  Demux1/1 -> Mux1/2, Gain2/1  "ax"
  Gain2/1 -> Mux/3
  Sum1/1 -> om_B/1  "om_B"
  Reshape/1 -> MatrixMultiply3/1
  Constant/1 -> Mux/2
  Mux/1 -> Mux3/2
  MatrixMultiply3/1 -> Sum1/2
  Demux1/2 -> Mux2/3, Gain3/1  "ay"
  Constant3/1 -> MatrixMultiply3/2
  Demux1/3 -> Gain1/1, Mux/1  "az"
  Mux1/1 -> Mux3/3
  Gain3/1 -> Mux1/1
  Mux3/1 -> Reshape/1
  Constant2/1 -> Mux1/3
  Gain1/1 -> Mux2/2
  Mux2/1 -> Mux3/1
  Demux/1 -> Mux4/1  "ax"
  Demux/2 -> Mux5/1  "ax_dot"
  Demux/3 -> Mux4/2  "ay"
  Demux/4 -> Mux5/2  "ay_dot"
  Demux/5 -> Mux4/3  "az"
  Demux/6 -> Mux5/3  "az_dot"
  alpha/1 -> Demux/1
  Mux4/1 -> Demux1/1
  Mux5/1 -> Sum1/1

== system kde/Subsystem/Actuator/state observer/Subsystem1 ==
  alpha : Inport
  A : Inport  Port=2
  C : Inport  Port=3
  B : Inport  Port=4
  MatrixMultiply : Product  Multiplication=Matrix(*)
  MatrixMultiply3 : Product  Multiplication=Matrix(*)
  Subsystem3 : Subsystem
  Sum1 : Sum  Inputs=|+-
  L : Outport
  A_hat*alpha : Outport  Port=2
  wires:
  A/1 -> Subsystem3/2(A), Sum1/1
  Sum1/1 -> MatrixMultiply/1  "A_hat"
  Subsystem3/1(L) -> MatrixMultiply3/1, L/1  "L"
  C/1 -> Subsystem3/3(C), MatrixMultiply3/2
  MatrixMultiply/1 -> A_hat*alpha/1  "A_hat*alpha"
  MatrixMultiply3/1 -> Sum1/2
  alpha/1 -> MatrixMultiply/2
  B/1 -> Subsystem3/1(B)

== system kde/Subsystem/Attitude Determination/Subsystem2/Subsystem ==
  Constant7 : Constant
  Constant8 : Constant
  Cos : Trigonometry  Operator=cos
  Cos1 : Trigonometry  Operator=cos
  Cos2 : Trigonometry  Operator=cos
  Mux : Mux  Inputs=3
  Product{,1,3..5} (5 alike) : Product
  Product2 : Product  Inputs=*/
  Sin : Trigonometry
  Sin1 : Trigonometry
  Square : Math  Operator=square
  Sum : Sum  Inputs=|++
  Sum1 : Sum  Inputs=|-+
  eccentricity : Constant  Value=orbit_E.e
  inclination : Constant  Value=orbit_E.inc
  semimajor axis : Constant  Value=orbit_E.a
  true anomaly : Subsystem
  R_N : Outport
  wires:
  Mux/1 -> Product5/2
  Product2/1 -> Product5/1  "earth distance magnitude"
  Product1/1 -> Product2/1
  Constant8/1 -> Sum1/2
  Sin/1 -> Product3/1, Product4/1
  true anomaly/1(theta) -> Sin/1, Cos1/1, Cos/1
  Cos/1 -> Product/2
  eccentricity/1 -> Product/1, Square/1
  Sin1/1 -> Product4/2
  Sum1/1 -> Product1/1
  Sum/1 -> Product2/2
  Product3/1 -> Mux/2
  Cos1/1 -> Mux/1
  Square/1 -> Sum1/1
  semimajor axis/1 -> Product1/2
  inclination/1 -> Sin1/1, Cos2/1
  Product4/1 -> Mux/3
  Constant7/1 -> Sum/2
  Product/1 -> Sum/1
  Product5/1 -> R_N/1
  Cos2/1 -> Product3/2

== system kde/Subsystem/Attitude Determination/Subsystem2/Subsystem1 ==
  alpha : Inport
  Constant : Constant
  Constant1 : Constant
  Constant2 : Constant
  Gain : Gain  Gain=-1
  Gain1 : Gain  Gain=-1
  Mux : Mux  Inputs=9
  Reshape : Reshape  OutputDimensionality=Customize  OutputDimensions=[3, 3]
  A_eps : Outport
  wires:
  Mux/1 -> Reshape/1
  Reshape/1 -> A_eps/1
  Constant/1 -> Mux/1
  Constant1/1 -> Mux/5
  Constant2/1 -> Mux/9
  alpha/1 -> Mux/7, Mux/6, Gain1/1, Gain/1, Mux/2
  Gain/1 -> Mux/4, Mux/3
  Gain1/1 -> Mux/8

== system kde/Subsystem/Attitude Determination/Subsystem2/Subsystem3 ==
  alpha : Inport
  Constant : Constant
  Constant1 : Constant
  Constant2 : Constant
  Gain : Gain  Gain=-1
  Gain1 : Gain  Gain=-1
  Mux : Mux  Inputs=9
  Reshape : Reshape  OutputDimensionality=Customize  OutputDimensions=[3, 3]
  A_eps : Outport
  wires:
  Mux/1 -> Reshape/1
  Reshape/1 -> A_eps/1
  Constant/1 -> Mux/1
  Constant1/1 -> Mux/5
  Constant2/1 -> Mux/9
  alpha/1 -> Mux/7, Mux/6, Gain1/1, Gain/1, Mux/2
  Gain/1 -> Mux/4, Mux/3
  Gain1/1 -> Mux/8

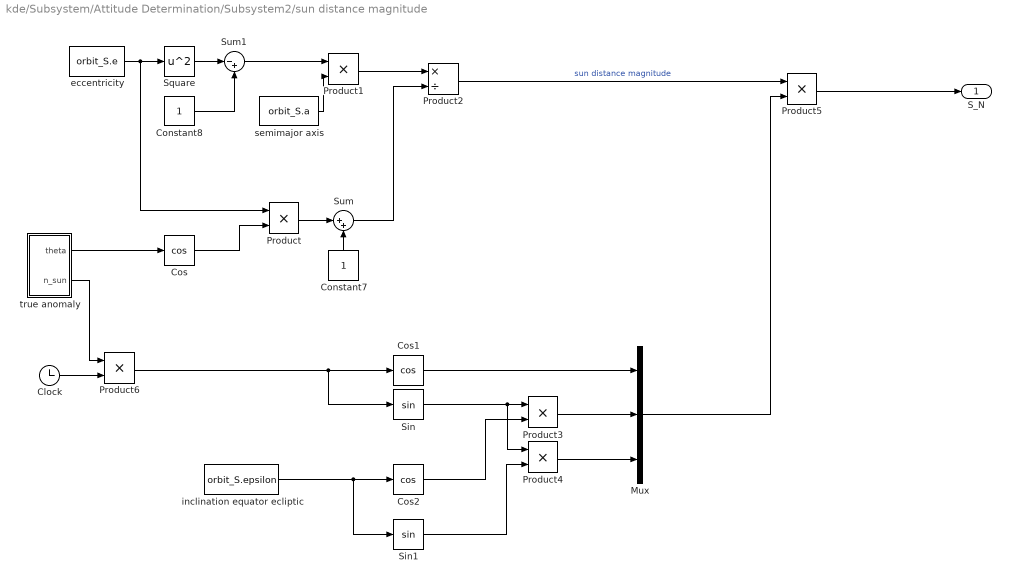
== system kde/Subsystem/Attitude Determination/Subsystem2/sun distance magnitude ==
  Clock : Clock
  Constant7 : Constant
  Constant8 : Constant
  Cos : Trigonometry  Operator=cos
  Cos1 : Trigonometry  Operator=cos
  Cos2 : Trigonometry  Operator=cos
  Mux : Mux  Inputs=3
  Product{,1,3..6} (6 alike) : Product
  Product2 : Product  Inputs=*/
  Sin : Trigonometry
  Sin1 : Trigonometry
  Square : Math  Operator=square
  Sum : Sum  Inputs=|++
  Sum1 : Sum  Inputs=|-+
  eccentricity : Constant  Value=orbit_S.e
  inclination equator ecliptic : Constant  Value=orbit_S.epsilon
  semimajor axis : Constant  Value=orbit_S.a
  true anomaly : Subsystem
  S_N : Outport
  wires:
  Mux/1 -> Product5/2
  Product2/1 -> Product5/1  "sun distance magnitude"
  Product1/1 -> Product2/1
  Constant8/1 -> Sum1/2
  Sin/1 -> Product4/1, Product3/1
  Cos/1 -> Product/2
  eccentricity/1 -> Product/1, Square/1
  Sin1/1 -> Product4/2
  Sum1/1 -> Product1/1
  Product3/1 -> Mux/2
  Cos1/1 -> Mux/1
  Square/1 -> Sum1/1
  semimajor axis/1 -> Product1/2
  inclination equator ecliptic/1 -> Sin1/1, Cos2/1
  Product4/1 -> Mux/3
  Constant7/1 -> Sum/2
  Product/1 -> Sum/1
  Cos2/1 -> Product3/2
  true anomaly/1(theta) -> Cos/1
  Clock/1 -> Product6/2
  true anomaly/2(n_sun) -> Product6/1
  Product6/1 -> Sin/1, Cos1/1
  Sum/1 -> Product2/2
  Product5/1 -> S_N/1

== system kde/Environment/Magnetic field/Magnetic field/Subsystem/true anomaly ==
  Constant : Constant  Value=orbit_E.theta0
  Constant1 : Constant  Value=orbit_E.n
  Constant10 : Constant  Value=3/2
  Constant8 : Constant
  Constant9 : Constant
  Cos : Trigonometry  Operator=cos
  Integrator : Integrator  InitialConditionSource=external
  Power : Math  Operator=pow
  Product1 : Product
  Product2 : Product
  Product3 : Product  Inputs=*/
  Square : Math  Operator=square
  Square1 : Math  Operator=square
  Sum : Sum  Inputs=|++
  Sum1 : Sum  Inputs=|-+
  eccentricity : Constant  Value=orbit_E.e
  theta : Outport
  wires:
  eccentricity/1 -> Square1/1, Product1/2
  Sum1/1 -> Power/1
  Product3/1 -> Integrator/1  "theta_dot"
  Constant9/1 -> Sum1/2
  Constant8/1 -> Sum/2
  Square1/1 -> Sum1/1
  Square/1 -> Product2/1
  Sum/1 -> Square/1
  Product2/1 -> Product3/1
  Cos/1 -> Product1/1
  Power/1 -> Product3/2
  Constant10/1 -> Power/2
  Integrator/1 -> theta/1, Cos/1  "theta"
  Constant/1 -> Integrator/2
  Product1/1 -> Sum/1
  Constant1/1 -> Product2/2

== system kde/Environment/air drag/air drag/Subsystem1/Subsystem ==
  Inc : Inport
  theta : Inport  Port=2
  Cos : Trigonometry  Operator=cos
  Cos1 : Trigonometry  Operator=cos
  Mux : Mux  Inputs=3
  Product1 : Product
  Product2 : Product
  Sin : Trigonometry
  Sin1 : Trigonometry
  Out1 : Outport
  wires:
  Sin1/1 -> Product2/1  "sin i"
  Cos/1 -> Mux/1  "cos  theta"
  Product1/1 -> Mux/2
  Sin/1 -> Product1/2, Product2/2  "sin theta"
  Product2/1 -> Mux/3
  Inc/1 -> Sin1/1, Cos1/1
  theta/1 -> Sin/1, Cos/1
  Cos1/1 -> Product1/1  "cos i"
  Mux/1 -> Out1/1

== system kde/Environment/air drag/air drag/Subsystem11/orientation s//c and solar panels ==
  Vector Concatenate : Concatenate  NumInputs=10  Mode=Multidimensional array  ConcatenateDimension=2
  orientation s/c and solar panels in B : Subsystem
  N_B : Outport
  wires:
  orientation s/c and solar panels in B/5(n5) -> Vector Concatenate/5
  orientation s/c and solar panels in B/7(n7) -> Vector Concatenate/7
  Vector Concatenate/1 -> N_B/1  "N_B"
  orientation s/c and solar panels in B/9(n9) -> Vector Concatenate/9
  orientation s/c and solar panels in B/3(n3) -> Vector Concatenate/3
  orientation s/c and solar panels in B/8(n8) -> Vector Concatenate/8
  orientation s/c and solar panels in B/10(n10) -> Vector Concatenate/10
  orientation s/c and solar panels in B/6(n6) -> Vector Concatenate/6
  orientation s/c and solar panels in B/2(n2) -> Vector Concatenate/2
  orientation s/c and solar panels in B/1(n1) -> Vector Concatenate/1
  orientation s/c and solar panels in B/4(n4) -> Vector Concatenate/4
